simulink model "ch7example28"  (Simulink 5.0)
settings: Solver=ode45  StartTime=0.0  StopTime=1000.0  FixedStep=1e-6  RelTol=1e-5
undefined symbols (not defined in the file): Fs
libraries: commdigbbndfm2 x4, dspsnks4 x4, commchan2 x1, commrandsrc2 x1, commsink2 x1, dspsigops x1, commutil2 x1, dspsigattribs x1, commseqgen2 x1
settings Model: LastModifiedBy=shaoyubin

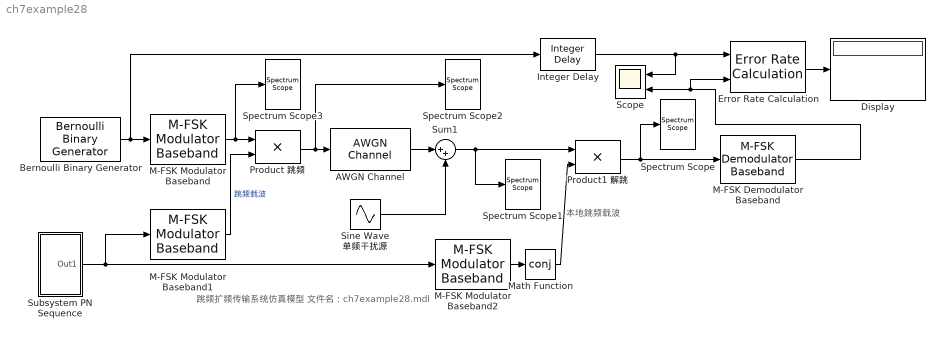
== system ch7example28 ==
  note: 跳频扩频传输系统仿真模型
      | 文件名：ch7example28.mdl
  note: 本地跳频载波
  AWGN Channel : commchan2/AWGN Channel  seed=67  noiseMode=Variance from mask  EsNodB=10  SNRdB=10  Ps=1  Tsym=1  variance=1
  Bernoulli Binary Generator : commrandsrc2/Bernoulli Binary Generator  P=0.5  seed=61  Ts=1/100  frameBased=off  sampPerFrame=1  orient=off
  Display : Display
  Error Rate Calculation : commsink2/Error Rate Calculation  N=0  st_delay=0  cp_mode=Entire frame  subframe=[]  PMode=Port  WsName=ErrorVec  RsMode2=off  stop=off  numErr=100  maxBits=1e6
  Integer Delay : dspsigops/Integer Delay  delay=1  ic=0  reset_popup=None
  M-FSK Demodulator Baseband : commdigbbndfm2/M-FSK Demodulator Baseband  M=2  OutType=Bit  Dec=Binary  freqSep=100  numSamp=40
  M-FSK Modulator Baseband : commdigbbndfm2/M-FSK Modulator Baseband  M=2  InType=Bit  Enc=Binary  freqSep=100  phaseType=Discontinuous  numSamp=40
  M-FSK Modulator Baseband1 : commdigbbndfm2/M-FSK Modulator Baseband  M=32  InType=Integer  Enc=Binary  freqSep=50  phaseType=Continuous  numSamp=80
  M-FSK Modulator Baseband2 : commdigbbndfm2/M-FSK Modulator Baseband  M=32  InType=Integer  Enc=Binary  freqSep=50  phaseType=Discontinuous  numSamp=80
  Math Function : Math  Operator=conj
  Product 跳频 : Product  SaturateOnIntegerOverflow=on
  Product1 解跳 : Product  SaturateOnIntegerOverflow=on
  Scope : Scope  NumInputPorts=2
      settings: TimeRange=0.2  YMin=-5~-5  YMax=5~5
  Sine Wave 单频干扰源 : Sin  Frequency=2*pi*150  SampleTime=1/4000
  Spectrum Scope : dspsnks4/Spectrum Scope  ScopeProperties=on  Domain=Frequency  HorizSpan=1  UseBuffer=on  BufferSize=1024  Overlap=0  inpFftLenInherit=on  FFTlength=1024  numAvg=500  DisplayProperties=off  AxisGrid=on  Memory=off  FrameNumber=on  AxisLegend=off  AxisZoom=off  OpenScopeAtSimStart=on  OpenScopeImmediately=off  FigPos=[232 258 560 420]  AxisProperties=off  XUnits=Hertz  XRange=[-Fs/2...Fs/2]  InheritXIncr=on  XIncr=1  XLabel=Samples  YUnits=dB  YLabel=Magnitude, dB  LineProperties=off  LineDisables=on|on|off|on  LineMarkers=|None  LineColors=|[1 0 0]
      settings: YMin=-70.2848426195927  YMax=23.5700499965559
  Spectrum Scope1 : dspsnks4/Spectrum Scope  ScopeProperties=off  Domain=Frequency  HorizSpan=1  UseBuffer=on  BufferSize=1024  Overlap=0  inpFftLenInherit=on  FFTlength=1024  numAvg=500  DisplayProperties=off  AxisGrid=on  Memory=off  FrameNumber=off  AxisLegend=off  AxisZoom=off  OpenScopeAtSimStart=on  OpenScopeImmediately=off  FigPos=[232 258 560 420]  AxisProperties=on  XUnits=Hertz  XRange=[-Fs/2...Fs/2]  InheritXIncr=on  XIncr=1  XLabel=Samples  YUnits=dB  YLabel=Magnitude, dB  LineProperties=off  LineDisables=off|off|on|off  LineMarkers=|None  LineColors=|[0 0 0]
      settings: YMin=-10  YMax=23.5700499965559
  Spectrum Scope2 : dspsnks4/Spectrum Scope  ScopeProperties=off  Domain=Frequency  HorizSpan=1  UseBuffer=on  BufferSize=1024  Overlap=0  inpFftLenInherit=on  FFTlength=1024  numAvg=500  DisplayProperties=off  AxisGrid=on  Memory=off  FrameNumber=off  AxisLegend=off  AxisZoom=off  OpenScopeAtSimStart=on  OpenScopeImmediately=off  FigPos=[232 258 560 420]  AxisProperties=on  XUnits=Hertz  XRange=[-Fs/2...Fs/2]  InheritXIncr=on  XIncr=1  XLabel=Samples  YUnits=dB  YLabel=Magnitude, dB  LineProperties=off  LineDisables=off|off|on|off  LineMarkers=|None  LineColors=|[0 0 0]
      settings: YMin=-10  YMax=23.5700499965559
  Spectrum Scope3 : dspsnks4/Spectrum Scope  ScopeProperties=off  Domain=Frequency  HorizSpan=1  UseBuffer=on  BufferSize=1024  Overlap=0  inpFftLenInherit=on  FFTlength=1024  numAvg=500  DisplayProperties=off  AxisGrid=on  Memory=off  FrameNumber=off  AxisLegend=off  AxisZoom=off  OpenScopeAtSimStart=on  OpenScopeImmediately=off  FigPos=[232 258 560 420]  AxisProperties=on  XUnits=Hertz  XRange=[-Fs/2...Fs/2]  InheritXIncr=on  XIncr=1  XLabel=Samples  YUnits=dB  YLabel=Magnitude, dB  LineProperties=off  LineDisables=off|off|on|off  LineMarkers=|None  LineColors=|[0 0 0]
      settings: YMin=-10  YMax=23.5700499965559
  "Subsystem PN Sequence " : Subsystem
  Sum1 : Sum  Inputs=|++  SaturateOnIntegerOverflow=on
  wires:
  Bernoulli Binary Generator/1 -> M-FSK Modulator Baseband/1, Integer Delay/1
  M-FSK Modulator Baseband/1 -> Product 跳频/1, Spectrum Scope3/1
  M-FSK Modulator Baseband1/1 -> Product 跳频/2  "跳频载波"
  "Subsystem PN Sequence "/1(Out1) -> M-FSK Modulator Baseband1/1, M-FSK Modulator Baseband2/1
  Product 跳频/1 -> AWGN Channel/1, Spectrum Scope2/1
  Math Function/1 -> Product1 解跳/2
  Product1 解跳/1 -> M-FSK Demodulator Baseband/1, Spectrum Scope/1
  M-FSK Modulator Baseband2/1 -> Math Function/1
  M-FSK Demodulator Baseband/1 -> Error Rate Calculation/2, Scope/2
  Error Rate Calculation/1 -> Display/1
  Sine Wave 单频干扰源/1 -> Sum1/2
  AWGN Channel/1 -> Sum1/1
  Sum1/1 -> Product1 解跳/1, Spectrum Scope1/1
  Integer Delay/1 -> Error Rate Calculation/1, Scope/1

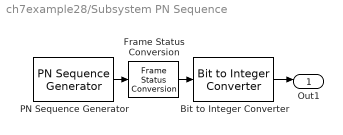
== system ch7example28/Subsystem PN Sequence  ==
  Bit to Integer Converter : commutil2/Bit to Integer Converter  nbits=5
  Frame Status Conversion : dspsigattribs/Frame Status Conversion  growRefPort=off  outframe=Sample-based
  PN Sequence Generator : commseqgen2/PN Sequence Generator  poly=[1 0 0 0 0 1 1]  ini_sta=[0 0 0 0 0 1]  shift=0  Ts=1/250  frameBased=on  sampPerFrame=5  reset=off
  Out1 : Outport
  wires:
  PN Sequence Generator/1 -> Frame Status Conversion/1
  Bit to Integer Converter/1 -> Out1/1
  Frame Status Conversion/1 -> Bit to Integer Converter/1
